simulink model "Simulation_FinalProject"  (R2024a)
settings: Solver=VariableStepAuto  StartTime=0.0  StopTime=100  RelTol=1e-3
undefined symbols (not defined in the file): K, L
settings Model: Creator=Hello  LastModifiedBy=mmelhanafy42
settings DebuggingCC: UnconnectedInputMsg=warning  UnconnectedOutputMsg=warning  UnconnectedLineMsg=warning
settings ModelReferenceCC: EnableRefExpFcnMdlSchedulingChecks=on
settings RTWCC: GPUComputeCapability=3.5  DLArmComputeVersion=19.05

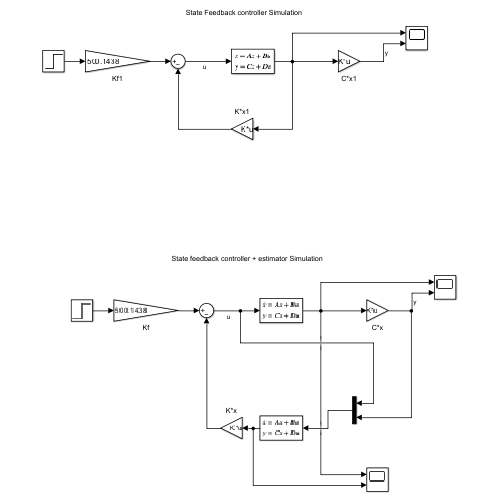
[thumbnail: Simulink's stored preview of the top-level diagram]
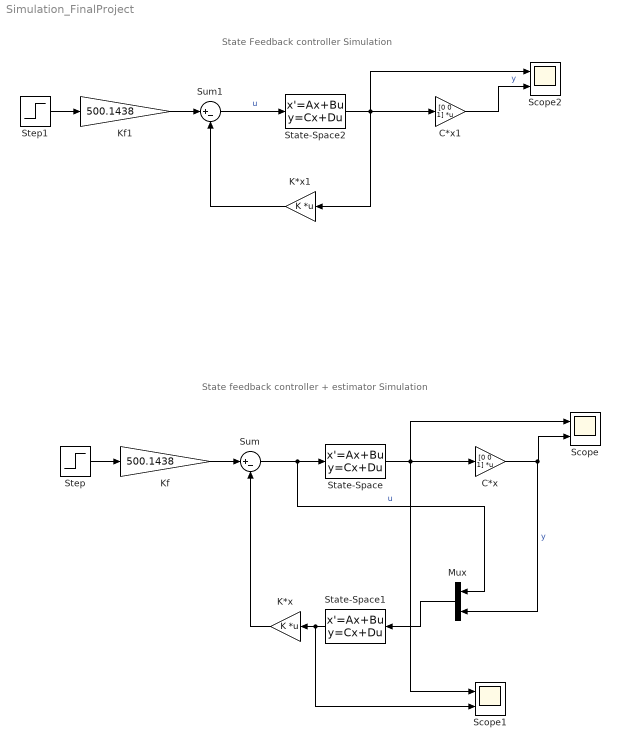
== system Simulation_FinalProject ==
  note: State Feedback controller Simulation
  note: State feedback controller + estimator Simulation
  C*x : Gain  Gain=[0 0 1]  Multiplication=Matrix(K*u)
  C*x1 : Gain  Gain=[0 0 1]  Multiplication=Matrix(K*u)
  K*x : Gain  Gain=K  Multiplication=Matrix(K*u)
  K*x1 : Gain  Gain=K  Multiplication=Matrix(K*u)
  Kf : Gain  Gain=500.1438
  Kf1 : Gain  Gain=500.1438
  Mux : Mux  Inputs=2
  Scope : Scope  NumInputPorts=2
  Scope1 : Scope  NumInputPorts=2
  Scope2 : Scope  NumInputPorts=2
  State-Space : StateSpace  A=[-0.313 56.7 0;-0.0139 -0.426 -5;0 56.7 0]  B=[0.232; 0.0203; 0]  C=eye(3)  D=zeros(3,1)  InitialCondition=0
  State-Space1 : StateSpace  A=[-0.313 56.7 0;-0.0139 -0.426 -5;0 56.7 0]-L*[0 0 1]  B=[0.232 L(1); 0.0203 L(2); 0 L(3)]  C=eye(3)  D=zeros(3,2)  InitialCondition=0
  State-Space2 : StateSpace  A=[-0.313 56.7 0;-0.0139 -0.426 -5;0 56.7 0]  B=[0.232; 0.0203; 0]  C=eye(3)  D=zeros(3,1)  InitialCondition=0
  Step : Step  Time=50  Before=1  After=2  SampleTime=0
  Step1 : Step  Time=50  Before=1  After=2  SampleTime=0
  Sum : Sum  Inputs=|+-
  Sum1 : Sum  Inputs=|+-
  wires:
  Sum/1 -> Mux/1, State-Space/1  "u"
  Kf/1 -> Sum/1
  Step/1 -> Kf/1
  State-Space/1 -> Scope1/1, C*x/1, Scope/1
  C*x/1 -> Mux/2, Scope/2  "y"
  K*x/1 -> Sum/2
  Mux/1 -> State-Space1/1
  State-Space1/1 -> Scope1/2, K*x/1
  K*x1/1 -> Sum1/2
  C*x1/1 -> Scope2/2  "y"
  State-Space2/1 -> K*x1/1, Scope2/1, C*x1/1
  Step1/1 -> Kf1/1
  Kf1/1 -> Sum1/1
  Sum1/1 -> State-Space2/1  "u"
